simulink model "diagrama3"  (R2024b)
settings: Solver=VariableStepAuto  StartTime=0.0  StopTime=0.5  RelTol=1e-3
values from neighbouring files (symbols this model uses):
  B1 = 0.001    [untitled.m]
  B2 = 0.001    [untitled.m]
  C1 = 0.001    [untitled.m]
  C2 = 0.001    [untitled.m]
undefined symbols (not defined in the file or in its folder): A, A1, A10, A11, A2, A3, A4, A5, A6, A7, A8, A9, B, B10, B11, B3, B4, B5, B6, B7, B8, B9, C, C10, C11, C3, C4, C5, C6, C7, C8, C9, D, D1, D10, D11, D2, D3, D4, D5, D6, D7, D8, D9
settings Model: Creator=Iustin  LastModifiedBy=Iustin

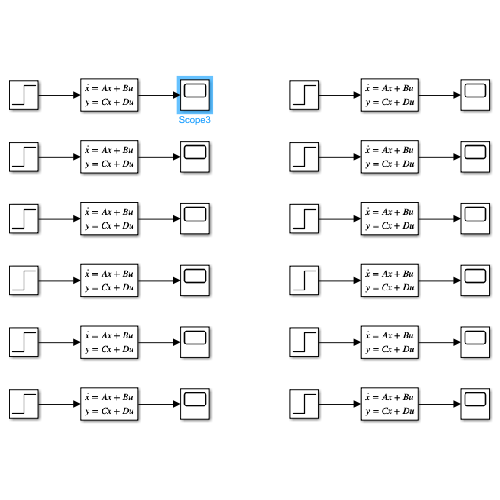
[thumbnail: Simulink's stored preview of the top-level diagram]
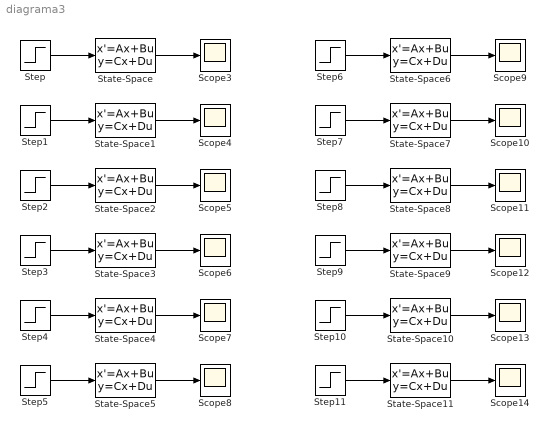
== system diagrama3 ==
  Scope{3..14} (12 alike) : Scope
  State-Space : StateSpace  A=A  B=B  C=C  D=D  InitialCondition=0
  State-Space1 : StateSpace  A=A1  B=B1  C=C1  D=D1  InitialCondition=0
  State-Space10 : StateSpace  A=A10  B=B10  C=C10  D=D10  InitialCondition=0
  State-Space11 : StateSpace  A=A11  B=B11  C=C11  D=D11  InitialCondition=0
  State-Space2 : StateSpace  A=A2  B=B2  C=C2  D=D2  InitialCondition=0
  State-Space3 : StateSpace  A=A3  B=B3  C=C3  D=D3  InitialCondition=0
  State-Space4 : StateSpace  A=A4  B=B4  C=C4  D=D4  InitialCondition=0
  State-Space5 : StateSpace  A=A5  B=B5  C=C5  D=D5  InitialCondition=0
  State-Space6 : StateSpace  A=A6  B=B6  C=C6  D=D6  InitialCondition=0
  State-Space7 : StateSpace  A=A7  B=B7  C=C7  D=D7  InitialCondition=0
  State-Space8 : StateSpace  A=A8  B=B8  C=C8  D=D8  InitialCondition=0
  State-Space9 : StateSpace  A=A9  B=B9  C=C9  D=D9  InitialCondition=0
  Step : Step  Time=0  After=0.1  SampleTime=0
  Step1 : Step  Time=0  After=0.2  SampleTime=0
  Step10 : Step  Time=0  After=1.1  SampleTime=0
  Step11 : Step  Time=0  After=1.2  SampleTime=0
  Step2 : Step  Time=0  After=0.3  SampleTime=0
  Step3 : Step  Time=0  After=0.4  SampleTime=0
  Step4 : Step  Time=0  After=0.5  SampleTime=0
  Step5 : Step  Time=0  After=0.6  SampleTime=0
  Step6 : Step  Time=0  After=0.7  SampleTime=0
  Step7 : Step  Time=0  After=0.8  SampleTime=0
  Step8 : Step  Time=0  After=0.9  SampleTime=0
  Step9 : Step  Time=0  SampleTime=0
  wires:
  State-Space10/1 -> Scope13/1
  Step3/1 -> State-Space3/1
  State-Space2/1 -> Scope5/1
  State-Space9/1 -> Scope12/1
  Step7/1 -> State-Space7/1
  State-Space11/1 -> Scope14/1
  Step6/1 -> State-Space6/1
  Step2/1 -> State-Space2/1
  State-Space8/1 -> Scope11/1
  Step4/1 -> State-Space4/1
  State-Space/1 -> Scope3/1
  Step10/1 -> State-Space10/1
  Step8/1 -> State-Space8/1
  State-Space7/1 -> Scope10/1
  Step1/1 -> State-Space1/1
  Step/1 -> State-Space/1
  State-Space5/1 -> Scope8/1
  State-Space4/1 -> Scope7/1
  Step11/1 -> State-Space11/1
  State-Space1/1 -> Scope4/1
  Step5/1 -> State-Space5/1
  Step9/1 -> State-Space9/1
  State-Space6/1 -> Scope9/1
  State-Space3/1 -> Scope6/1
